simulink model "halfadder"  (R2025b)
settings: Solver=VariableStepAuto  StartTime=0.0  StopTime=10.0  RelTol=1e-3
settings Model: Creator=cyber  LastModifiedBy=cyber

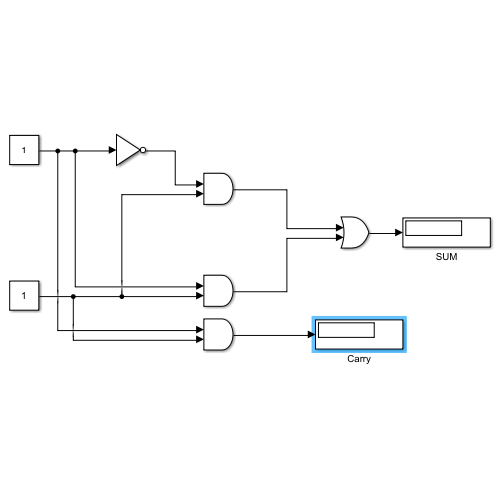
[thumbnail: Simulink's stored preview of the top-level diagram]
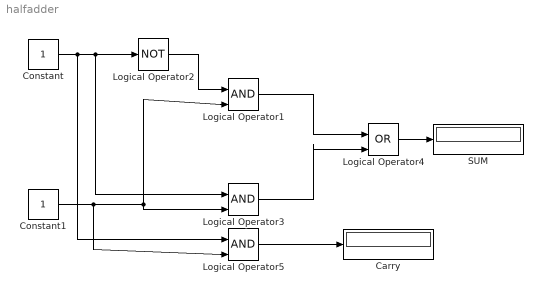
== system halfadder ==
  Carry : Display
  Constant : Constant
  Constant1 : Constant
  Logical Operator1 : Logic  IconShape=distinctive  AllPortsSameDT=off  OutDataTypeStr=boolean
  Logical Operator2 : Logic  Operator=NOT  IconShape=distinctive  AllPortsSameDT=off  OutDataTypeStr=boolean
  Logical Operator3 : Logic  IconShape=distinctive  AllPortsSameDT=off  OutDataTypeStr=boolean
  Logical Operator4 : Logic  Operator=OR  IconShape=distinctive  AllPortsSameDT=off  OutDataTypeStr=boolean
  Logical Operator5 : Logic  IconShape=distinctive  AllPortsSameDT=off  OutDataTypeStr=boolean
  SUM : Display
  wires:
  Constant/1 -> Logical Operator5/1, Logical Operator3/1, Logical Operator2/1
  Constant1/1 -> Logical Operator5/2, Logical Operator3/2, Logical Operator1/2
  Logical Operator2/1 -> Logical Operator1/1
  Logical Operator1/1 -> Logical Operator4/1
  Logical Operator3/1 -> Logical Operator4/2
  Logical Operator4/1 -> SUM/1
  Logical Operator5/1 -> Carry/1
